simulink model "HyTech_Simulink"  (R2019a)
settings: Solver=ode23t  StartTime=0.0  StopTime=Sch_Cycle(end,1)  RelTol=1e-3  EnableMultiTasking=on
InitFcn:
  | Vehicle_Init_File_L3
StopFcn:
  | Vehicle_Post_File
values from neighbouring files (symbols this model uses):
  Battery_Capacity = 5800/300    (= 19.3333333333)    [Vehicle_Init_File_L3.m]
  Battery_Initial_SOC = 0.9    [Vehicle_Init_File_L3.m]
  Battery_OCV_Data = [3.327826569 3.331337005 3.334822767 3.33828398 3.341720768 3.345133257 3.348521571 3.351885833 3.355226166 3.358542694 3.36183554 3.365104826 ... (412 elements, 1x412)]    [Battery_Data.mat]
  Battery_OCV_SOC_Axis = [0.0004004004004 0.001701701702 0.003003003003 0.004304304304 0.005605605606 0.006906906907 0.008208208208 0.00950950951 0.01081081081 0.01211211211 0.01341341341 0.01471471471 ... (412 elements, 1x412)]    [Battery_Data.mat]
  Battery_OCV_Temp_Axis = [0 10 20 35 55]    [Battery_Data.mat]
  Battery_R_Charge_Data = [1.20043849237 1.12672735687 1.10566703244 1.13725751908 1.18990833015 1.24255914122 1.32680043893 1.43210206107 1.52687352099 0.62127957061 0.5370382729 0.494917624045 ... (45 elements, 9x5)]    [Battery_Data.mat]
  Battery_R_Discharge_Data = [24.63444624 24.49083095 24.34792772 24.20573418 24.06424798 23.92346676 23.78338817 23.64400987 23.5053295 23.36734475 23.23005326 23.09345271 ... (412 elements, 1x412)]    [Battery_Data.mat]
  Battery_R_SOC_Axis = [0.0004004004004 0.001701701702 0.003003003003 0.004304304304 0.005605605606 0.006906906907 0.008208208208 0.00950950951 0.01081081081 0.01211211211 0.01341341341 0.01471471471 ... (412 elements, 1x412)]    [Battery_Data.mat]
  battery_soc_high = 0.9    [Vehicle_Init_File_L3.m]
  battery_soc_low = 0.1    [Vehicle_Init_File_L3.m]
  Front_Sprocket_Teeth = 8    [Vehicle_Init_File_L3.m]
  Logging_Sample_Time_s = 0.01    [Vehicle_Init_File_L3.m]
  Max_Current_Charge = 250    [Vehicle_Init_File_L3.m]
  Max_Current_Discharge = -250    [Vehicle_Init_File_L3.m]
  Rear_Sprocket_Teeth = 41    [Vehicle_Init_File_L3.m]
  Vehicle_Tire_Radius = 0.2286    [Vehicle_Init_File_L3.m]
undefined symbols (not defined in the file or in its folder): Battery_R_Temp_Axis, MG_Eff_Data, MG_Eff_RPM_Axis, MG_Eff_Torque_Axis, MG_Torque_Data, MG_Torque_RPM_Axis, Sch_Cycle
libraries: nesl_utility x12, fl_lib x10, sdl_lib x3, simulink x1
settings Model: Creator=sloghavi3  LastModifiedBy=mweist6
settings SolverCC: SolverResetMethod=Robust
settings DataIOCC: ReturnWorkspaceOutputs=off
settings OptimizationCC: LifeSpan=inf
settings DebuggingCC: PregeneratedLibrarySubsystemCodeDiagnostic=none  SFUnexpectedBacktrackingDiag=warning  SFNoUnconditionalDefaultTransitionDiag=warning  SFExecutionAtInitializationDiag=none  ArithmeticOperatorsInVariantConditions=warning
settings SFSimCC: SimUseLocalCustomCode=off
settings RTWCC: RTWUseLocalCustomCode=off
settings CodeAppCC: StateflowObjectComments=on
settings GRTTargetCC: TargetLangStandard=C89/C90 (ANSI)  GeneratePreprocessorConditionals=Disable all
settings ConfigComp: CovMetricSettings=dw  CovHtmlReporting=on  CovSaveCumulativeToWorkspaceVar=on  CovSaveSingleToWorkspaceVar=on  CovExternalEMLEnable=off
settings SimscapeCC: SimscapeNormalizeSystem=off

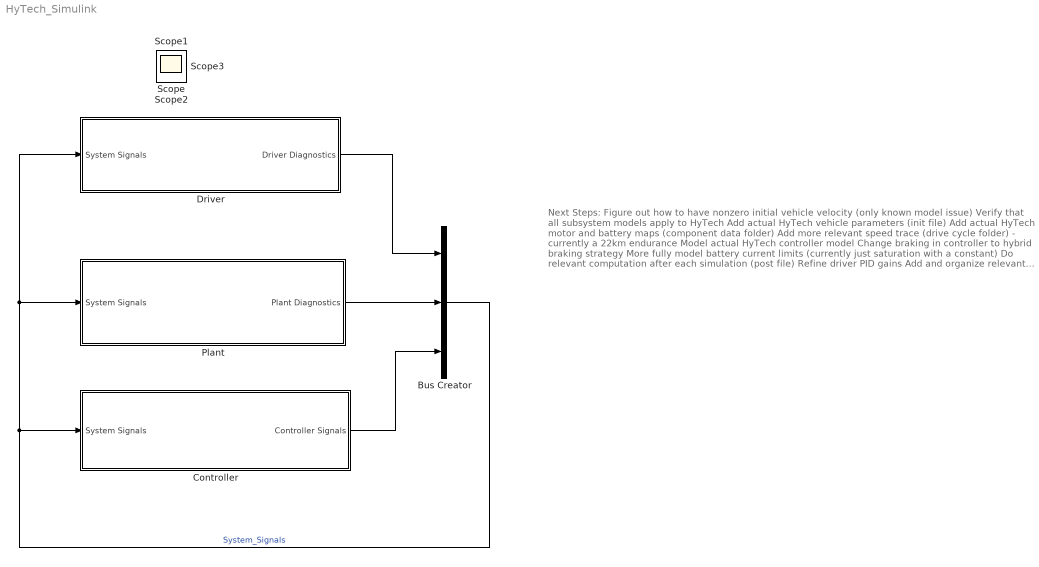
== system HyTech_Simulink ==
  note: Next Steps:
      |
      | Figure out how to have nonzero initial vehicle velocity (only known model issue)
      | Verify that all subsystem models apply to HyTech
      | Add actual HyTech vehicle parameters (init file)
      | Add actual HyTech motor and battery maps (component data folder)
      | Add more relevant speed trace (drive cycle folder) - currently a 22km endurance
      | Model actual HyTech controller model
      | Change braking in controller to hybrid braking strategy
      | More fully model battery current limits (currently just saturation with a constant)
      | Do relevant computation after each simulation (post file)
      | Refine driver PID gains
      | Add and organize relevant scopes in Logging and Visualization subsystem
  Bus Creator : BusCreator  Inputs=3
  Controller : Subsystem
  Driver : Subsystem
  Plant : Subsystem
  Scope{,1..3} (4 alike) : Scope
  wires:
  Driver/1(Driver Diagnostics) -> Bus Creator/1
  Plant/1(Plant Diagnostics) -> Bus Creator/2
  Controller/1(Controller Signals) -> Bus Creator/3
  Bus Creator/1 -> Driver/1(System Signals), Plant/1(System Signals), Controller/1(System Signals)  "System_Signals"

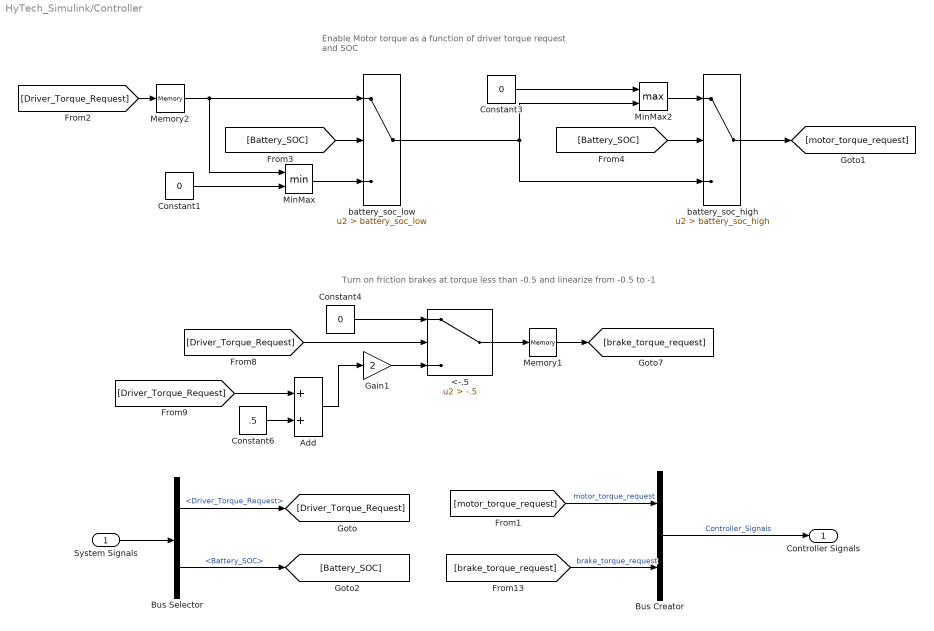
== system HyTech_Simulink/Controller ==
  note: Enable Motor torque as a function of driver torque request
      | and SOC
  note: Turn on friction brakes at torque less than -0.5 and linearize from -0.5 to -1
  System Signals : Inport
  <-.5 : Switch  Criteria=u2 > Threshold  Threshold=-.5
  Add : Sum
  Bus Creator : BusCreator  Inputs=2
  Bus Selector : BusSelector  OutputSignals=Driver_Diagnostics.Driver_Torque_Request,Plant_Diagnostics.Battery_Diagnostics.Battery_SOC
  Constant1 : Constant  Value=0
  Constant3 : Constant  Value=0
  Constant4 : Constant  Value=0
  Constant6 : Constant  Value=.5
  Gain1 : Gain  Gain=2
  Memory1 : Memory
  Memory2 : Memory
  MinMax : MinMax  Inputs=2
  MinMax2 : MinMax  Function=max  Inputs=2
  battery_soc_high : Switch  Criteria=u2 > Threshold  Threshold=battery_soc_high
  battery_soc_low : Switch  Criteria=u2 > Threshold  Threshold=battery_soc_low
  Controller Signals : Outport
  wires:
  Bus Creator/1 -> Controller Signals/1  "Controller_Signals"
  System Signals/1 -> Bus Selector/1
  Bus Selector/1 -> [Driver_Torque_Request]  "<Driver_Torque_Request>"
  [motor_torque_request] -> Bus Creator/1  "motor_torque_request"
  Bus Selector/2 -> [Battery_SOC]  "<Battery_SOC>"
  [Battery_SOC] -> battery_soc_low/2
  [Driver_Torque_Request] -> Memory2/1
  MinMax/1 -> battery_soc_low/3
  [Driver_Torque_Request] -> <-.5/2
  Constant4/1 -> <-.5/1
  [Driver_Torque_Request] -> Add/1
  Constant6/1 -> Add/2
  Add/1 -> Gain1/1
  Gain1/1 -> <-.5/3
  <-.5/1 -> Memory1/1
  [Battery_SOC] -> battery_soc_high/2
  [brake_torque_request] -> Bus Creator/2  "brake_torque_request"
  Memory1/1 -> [brake_torque_request]
  Constant1/1 -> MinMax/2
  battery_soc_low/1 -> battery_soc_high/3, MinMax2/2
  battery_soc_high/1 -> [motor_torque_request]
  Memory2/1 -> MinMax/1, battery_soc_low/1
  MinMax2/1 -> battery_soc_high/1
  Constant3/1 -> MinMax2/1

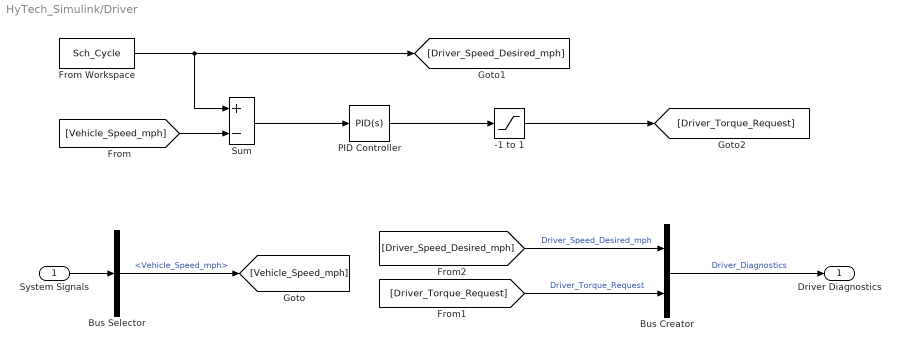
== system HyTech_Simulink/Driver ==
  System Signals : Inport
  -1 to 1 : Saturate  UpperLimit=1  LowerLimit=-1
  Bus Creator : BusCreator  Inputs=2
  Bus Selector : BusSelector  OutputSignals=Plant_Diagnostics.Vehicle_Diagnostics.Vehicle_Speed_mph
  From Workspace : FromWorkspace  VariableName=Sch_Cycle  SampleTime=0
  PID Controller : simulink/Continuous/PID Controller  Controller=PID  Form=Parallel  TimeDomain=Continuous-time  SampleTime=-1  IntegratorMethod=Forward Euler  FilterMethod=Forward Euler  ControllerParametersSource=internal  P=.5  I=.05  D=0.05  UseFilter=on  N=100  TunerSelectOption=Transfer Function Based (PID Tuner App)  InitialConditionSource=internal  InitialConditionForIntegrator=0  InitialConditionForFilter=0  DifferentiatorICPrevScaledInput=0  ExternalReset=none  TrackingMode=off  Kt=1  LimitOutput=off  UpperSaturationLimit=inf  LowerSaturationLimit=-inf  LinearizeAsGain=on  AntiWindupMode=none  Kb=1  POutMin=[]  POutMax=[]  IOutMin=[]  IOutMax=[]  DOutMin=[]  DOutMax=[]  NOutMin=[]  NOutMax=[]  SumOutMin=[]  SumOutMax=[]  SaturationOutMin=[]  SaturationOutMax=[]  PParamMin=[]  PParamMax=[]  IParamMin=[]  IParamMax=[]  DParamMin=[]  DParamMax=[]  NParamMin=[]  NParamMax=[]  KbParamMin=[]  KbParamMax=[]  KtParamMin=[]  KtParamMax=[]  KbOutMin=[]  KbOutMax=[]  KtOutMin=[]  KtOutMax=[]  IntegratorOutMin=[]  IntegratorOutMax=[]  FilterOutMin=[]  FilterOutMax=[]  SumI1OutMin=[]  SumI1OutMax=[]  SumI2OutMin=[]  SumI2OutMax=[]  SumI3OutMin=[]  SumI3OutMax=[]  SumI4OutMin=[]  SumI4OutMax=[]  SumDOutMin=[]  SumDOutMax=[]  DifferentiatorOutMin=[]  DifferentiatorOutMax=[]  FilterDiffOutCoefMin=[]  FilterDiffOutCoefMax=[]  ReciprocalOutMin=[]  ReciprocalOutMax=[]  SumDenOutMin=[]  SumDenOutMax=[]  SumNumOutMin=[]  SumNumOutMax=[]  DivideOutMin=[]  DivideOutMax=[]  IntegratorContinuousStateAttributes=''  IntegratorStateMustResolveToSignalObject=off  IntegratorRTWStateStorageClass=Auto  FilterContinuousStateAttributes=''  FilterStateMustResolveToSignalObject=off  FilterRTWStateStorageClass=Auto  ParallelPVariant=InternalParameters  IdealPVariant=Disabled  IVariant=InternalParameters  DVariant=InternalParameters  IntegratorVariant=Continuous  SatVariant=Disabled  AWVariant=Passthrough  PCopyVariant=Disabled  TRVariant=Disabled  FdbkBlocksVariant=Forward  IdealPFdbkVariant=Disabled  SatFdbkVariant=Disabled  DerivativeFilterVariant=ContFilter  NVariant=InternalParameters  NCopyVariant=Disabled  FilterICVariant=InternalICsFilter  IntegratorICVariant=InternalICs  ExternalResetVariant=Disabled  TRSumVariant=Passthrough  SumFdbkVariant=Disabled  SumVariant=Sum_PID
  Sum : Sum  Inputs=+-
  Driver Diagnostics : Outport
  wires:
  Bus Creator/1 -> Driver Diagnostics/1  "Driver_Diagnostics"
  System Signals/1 -> Bus Selector/1
  Bus Selector/1 -> [Vehicle_Speed_mph]  "<Vehicle_Speed_mph>"
  [Vehicle_Speed_mph] -> Sum/2
  From Workspace/1 -> [Driver_Speed_Desired_mph], Sum/1
  Sum/1 -> PID Controller/1
  PID Controller/1 -> -1 to 1/1
  -1 to 1/1 -> [Driver_Torque_Request]
  [Driver_Torque_Request] -> Bus Creator/2  "Driver_Torque_Request"
  [Driver_Speed_Desired_mph] -> Bus Creator/1  "Driver_Speed_Desired_mph"

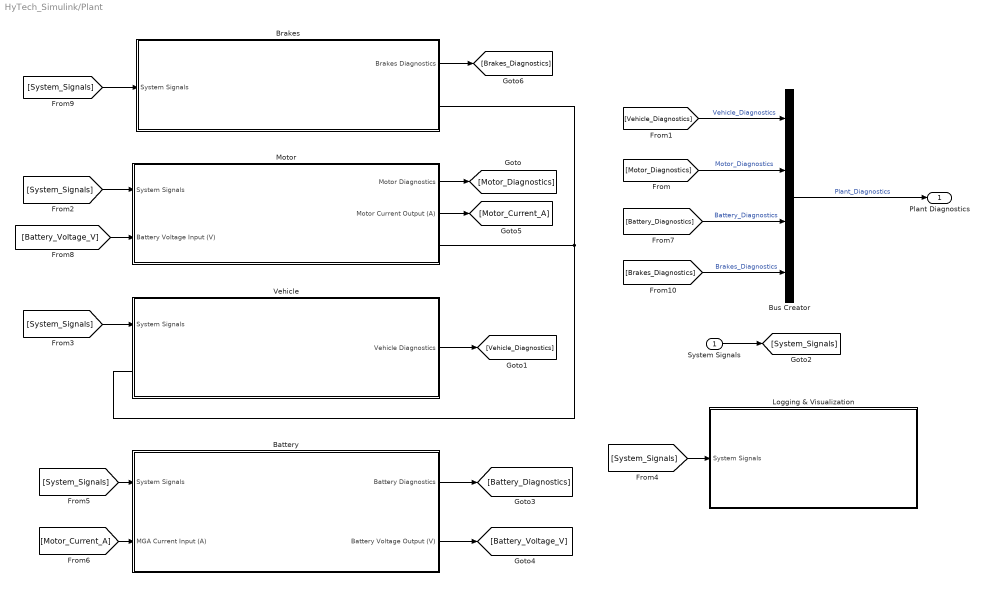
== system HyTech_Simulink/Plant ==
  System Signals : Inport
  Battery : Subsystem
  Brakes : Subsystem
  Bus Creator : BusCreator  Inputs=4
  Logging & Visualization : Subsystem
  Motor : Subsystem
  Vehicle : Subsystem
  Plant Diagnostics : Outport
  wires:
  Bus Creator/1 -> Plant Diagnostics/1  "Plant_Diagnostics"
  System Signals/1 -> [System_Signals]
  Motor/1(Motor Diagnostics) -> [Motor_Diagnostics]
  [Motor_Diagnostics] -> Bus Creator/2  "Motor_Diagnostics"
  [Vehicle_Diagnostics] -> Bus Creator/1  "Vehicle_Diagnostics"
  [System_Signals] -> Motor/1(System Signals)
  [System_Signals] -> Vehicle/1(System Signals)
  [System_Signals] -> Logging & Visualization/1(System Signals)
  [System_Signals] -> Battery/1(System Signals)
  Battery/2("Battery Voltage Output (V) ") -> [Battery_Voltage_V]
  Battery/1("Battery Diagnostics ") -> [Battery_Diagnostics]
  [Motor_Current_A] -> Battery/2("MGA Current Input (A) ")
  [Battery_Diagnostics] -> Bus Creator/3  "Battery_Diagnostics"
  Vehicle/1(Vehicle Diagnostics) -> [Vehicle_Diagnostics]
  [Battery_Voltage_V] -> Motor/2("Battery Voltage Input (V) ")
  Motor/2("Motor Current Output (A) ") -> [Motor_Current_A]
  [System_Signals] -> Brakes/1(System Signals)
  Brakes/1(Brakes Diagnostics) -> [Brakes_Diagnostics]
  [Brakes_Diagnostics] -> Bus Creator/4  "Brakes_Diagnostics"
  connections:
  Brakes/RConn1 -- Vehicle/LConn1 -- Motor/RConn1

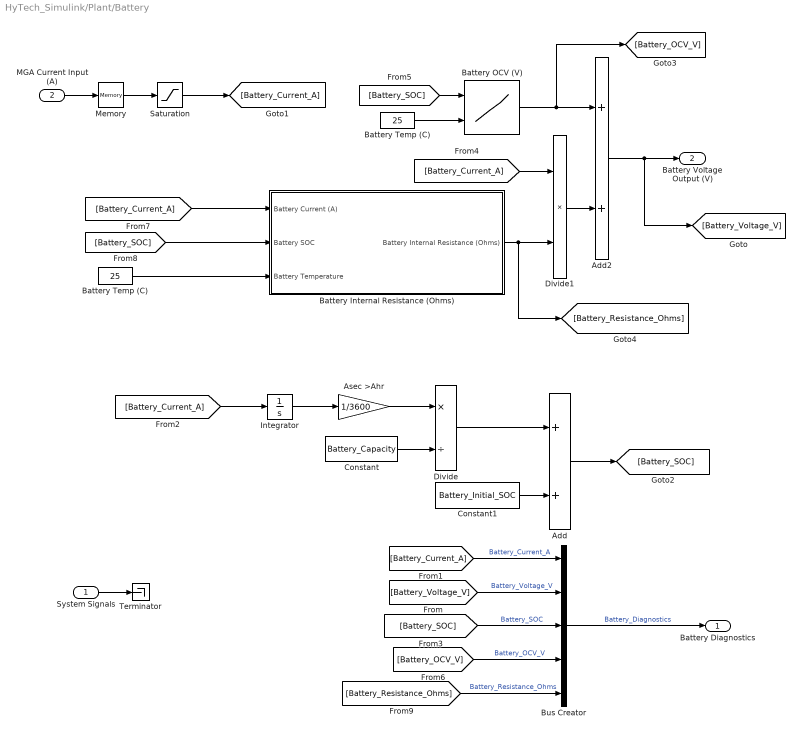
== system HyTech_Simulink/Plant/Battery ==
  System Signals : Inport
  "MGA Current Input (A) " : Inport  Port=2
  Add : Sum
  Add2 : Sum
  Asec >Ahr : Gain  Gain=1/3600
  "Battery Internal Resistance (Ohms) " : Subsystem
  Battery OCV (V) : Lookup_n-D  BreakpointsForDimension1=Battery_OCV_SOC_Axis  BreakpointsForDimension2=Battery_OCV_Temp_Axis  Table=Battery_OCV_Data  InternalRulePriority=Speed  RndMeth=Simplest  InputSameDT=on
  Battery Temp (C) : Constant  Value=25
  "Battery Temp (C) " : Constant  Value=25
  Bus Creator : BusCreator  Inputs=5
  Constant : Constant  Value=Battery_Capacity
  Constant1 : Constant  Value=Battery_Initial_SOC
  Divide : Product  Inputs=*/
  Divide1 : Product  Inputs=**
  Integrator : Integrator
  Memory : Memory
  Saturation : Saturate  UpperLimit=Max_Current_Charge  LowerLimit=Max_Current_Discharge
  Terminator : Terminator
  "Battery Diagnostics " : Outport
  "Battery Voltage Output (V) " : Outport  Port=2
  wires:
  System Signals/1 -> Terminator/1
  Bus Creator/1 -> "Battery Diagnostics "/1  "Battery_Diagnostics"
  [Battery_Voltage_V] -> Bus Creator/2  "Battery_Voltage_V"
  [Battery_Current_A] -> Bus Creator/1  "Battery_Current_A"
  [Battery_Current_A] -> Integrator/1
  Integrator/1 -> Asec >Ahr/1
  Asec >Ahr/1 -> Divide/1
  Constant/1 -> Divide/2
  Constant1/1 -> Add/2
  Divide/1 -> Add/1
  Add/1 -> [Battery_SOC]
  [Battery_SOC] -> Bus Creator/3  "Battery_SOC"
  "MGA Current Input (A) "/1 -> Memory/1
  [Battery_Current_A] -> Divide1/1
  Divide1/1 -> Add2/2
  Add2/1 -> [Battery_Voltage_V], "Battery Voltage Output (V) "/1
  Battery OCV (V)/1 -> [Battery_OCV_V], Add2/1
  "Battery Temp (C) "/1 -> Battery OCV (V)/2
  [Battery_SOC] -> Battery OCV (V)/1
  [Battery_OCV_V] -> Bus Creator/4  "Battery_OCV_V"
  "Battery Internal Resistance (Ohms) "/1("Battery Internal Resistance (Ohms) ") -> [Battery_Resistance_Ohms], Divide1/2
  [Battery_Current_A] -> "Battery Internal Resistance (Ohms) "/1(Battery Current (A))
  [Battery_SOC] -> "Battery Internal Resistance (Ohms) "/2(Battery SOC)
  Battery Temp (C)/1 -> "Battery Internal Resistance (Ohms) "/3("Battery Temperature ")
  [Battery_Resistance_Ohms] -> Bus Creator/5  "Battery_Resistance_Ohms"
  Memory/1 -> Saturation/1
  Saturation/1 -> [Battery_Current_A]

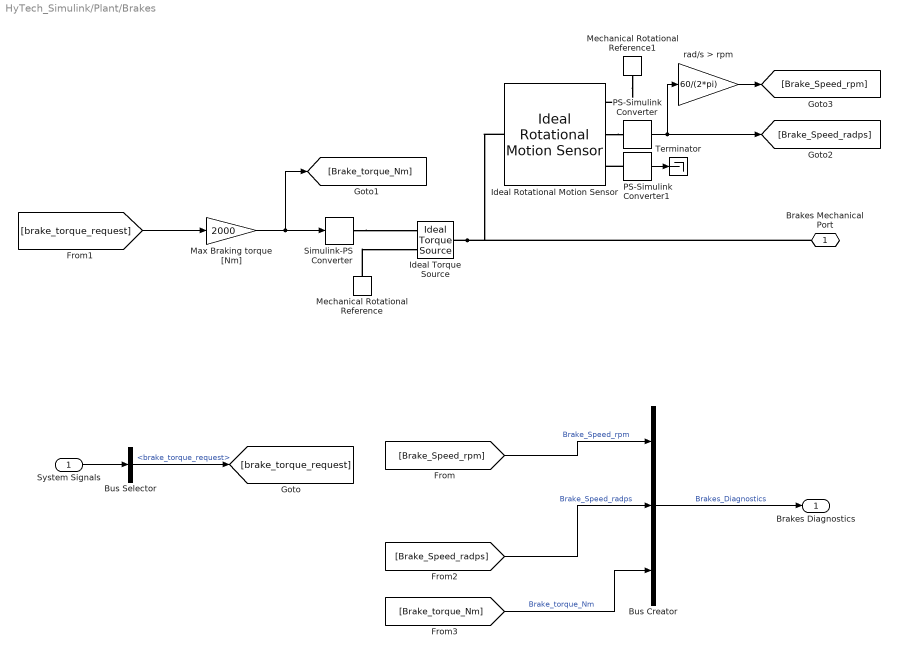
== system HyTech_Simulink/Plant/Brakes ==
  System Signals : Inport
  Bus Creator : BusCreator  Inputs=3
  Bus Selector : BusSelector  OutputSignals=Controller_Signals.brake_torque_request
  Ideal Rotational Motion Sensor : fl_lib/Mechanical/Mechanical Sensors/Ideal Rotational Motion Sensor  offset=0 rad
  Ideal Torque Source : fl_lib/Mechanical/Mechanical Sources/Ideal Torque Source
  Max Braking torque [Nm] : Gain  Gain=2000
  Mechanical Rotational Reference : fl_lib/Mechanical/Rotational Elements/Mechanical Rotational Reference
  Mechanical Rotational Reference1 : fl_lib/Mechanical/Rotational Elements/Mechanical Rotational Reference
  PS-Simulink Converter : nesl_utility/PS-Simulink Converter  PhysicalDomain=network_engine_domain  SubClassName=ps_output  LeftPortType=input  RightPortType=output  PseudoPeriodic=off  Frequencies=[]  Unit=1  AffineConversion=off
  PS-Simulink Converter1 : nesl_utility/PS-Simulink Converter  PhysicalDomain=network_engine_domain  SubClassName=ps_output  LeftPortType=input  RightPortType=output  PseudoPeriodic=off  Frequencies=[]  Unit=1  AffineConversion=off
  Simulink-PS Converter : nesl_utility/Simulink-PS Converter  PhysicalDomain=network_engine_domain  SubClassName=ps_input  LeftPortType=input  RightPortType=output  PseudoPeriodic=off  Frequencies=[]  NoiseDistribution=none  NoiseParameters=[]  Unit=1  AffineConversion=off  FilteringAndDerivatives=zero  SimscapeFilterOrder=2  InputFilterTimeConstant=0.01  UdotUserProvided=1
  Terminator : Terminator
  rad/s > rpm : Gain  Gain=60/(2*pi)
  Brakes Mechanical Port : PMIOPort  Side=Right
  Brakes Diagnostics : Outport
  wires:
  PS-Simulink Converter/1 -> rad/s > rpm/1, [Brake_Speed_radps]
  System Signals/1 -> Bus Selector/1
  PS-Simulink Converter1/1 -> Terminator/1
  rad/s > rpm/1 -> [Brake_Speed_rpm]
  Bus Selector/1 -> [brake_torque_request]  "<brake_torque_request>"
  [brake_torque_request] -> Max Braking torque [Nm]/1
  Bus Creator/1 -> Brakes Diagnostics/1  "Brakes_Diagnostics"
  [Brake_Speed_rpm] -> Bus Creator/1  "Brake_Speed_rpm"
  [Brake_Speed_radps] -> Bus Creator/2  "Brake_Speed_radps"
  Max Braking torque [Nm]/1 -> [Brake_torque_Nm], Simulink-PS Converter/1
  [Brake_torque_Nm] -> Bus Creator/3  "Brake_torque_Nm"
  connections:
  Ideal Torque Source/LConn1 -- Brakes Mechanical Port/RConn1 -- Ideal Rotational Motion Sensor/LConn1
  Simulink-PS Converter/RConn1 -- Ideal Torque Source/RConn1
  Mechanical Rotational Reference/LConn1 -- Ideal Torque Source/RConn2
  PS-Simulink Converter1/LConn1 -- Ideal Rotational Motion Sensor/RConn3
  Mechanical Rotational Reference1/LConn1 -- Ideal Rotational Motion Sensor/RConn1
  Ideal Rotational Motion Sensor/RConn2 -- PS-Simulink Converter/LConn1

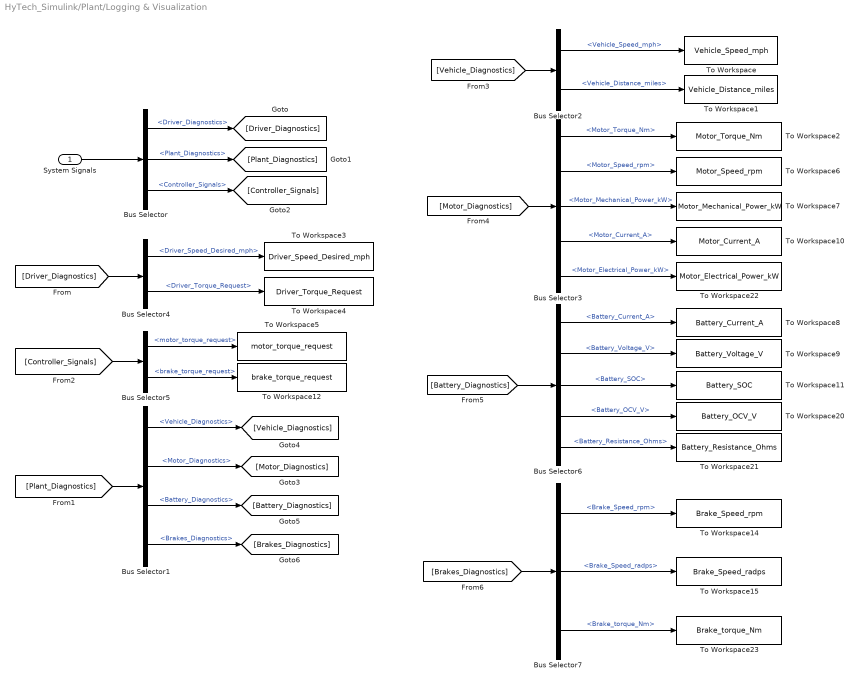
== system HyTech_Simulink/Plant/Logging & Visualization ==
  System Signals : Inport
  Bus Selector : BusSelector  OutputSignals=Driver_Diagnostics,Plant_Diagnostics,Controller_Signals
  Bus Selector1 : BusSelector  OutputSignals=Vehicle_Diagnostics,Motor_Diagnostics,Battery_Diagnostics,Brakes_Diagnostics
  Bus Selector2 : BusSelector  OutputSignals=Vehicle_Speed_mph,Vehicle_Distance_miles
  Bus Selector3 : BusSelector  OutputSignals=Motor_Torque_Nm,Motor_Speed_rpm,Motor_Mechanical_Power_kW,Motor_Current_A,Motor_Electrical_Power_kW
  Bus Selector4 : BusSelector  OutputSignals=Driver_Speed_Desired_mph,Driver_Torque_Request
  Bus Selector5 : BusSelector  OutputSignals=motor_torque_request,brake_torque_request
  Bus Selector6 : BusSelector  OutputSignals=Battery_Current_A,Battery_Voltage_V,Battery_SOC,Battery_OCV_V,Battery_Resistance_Ohms
  Bus Selector7 : BusSelector  OutputSignals=Brake_Speed_rpm,Brake_Speed_radps,Brake_torque_Nm
  To Workspace : ToWorkspace  VariableName=Vehicle_Speed_mph  SampleTime=Logging_Sample_Time_s
  To Workspace1 : ToWorkspace  VariableName=Vehicle_Distance_miles  SampleTime=Logging_Sample_Time_s
  To Workspace10 : ToWorkspace  VariableName=Motor_Current_A  SampleTime=Logging_Sample_Time_s
  To Workspace11 : ToWorkspace  VariableName=Battery_SOC  SampleTime=Logging_Sample_Time_s
  To Workspace12 : ToWorkspace  VariableName=brake_torque_request  SampleTime=Logging_Sample_Time_s
  To Workspace14 : ToWorkspace  VariableName=Brake_Speed_rpm  SampleTime=Logging_Sample_Time_s
  To Workspace15 : ToWorkspace  VariableName=Brake_Speed_radps  SampleTime=Logging_Sample_Time_s
  To Workspace2 : ToWorkspace  VariableName=Motor_Torque_Nm  SampleTime=Logging_Sample_Time_s
  To Workspace20 : ToWorkspace  VariableName=Battery_OCV_V  SampleTime=Logging_Sample_Time_s
  To Workspace21 : ToWorkspace  VariableName=Battery_Resistance_Ohms  SampleTime=Logging_Sample_Time_s
  To Workspace22 : ToWorkspace  VariableName=Motor_Electrical_Power_kW  SampleTime=Logging_Sample_Time_s
  To Workspace23 : ToWorkspace  VariableName=Brake_torque_Nm  SampleTime=Logging_Sample_Time_s
  To Workspace3 : ToWorkspace  VariableName=Driver_Speed_Desired_mph  SampleTime=Logging_Sample_Time_s
  To Workspace4 : ToWorkspace  VariableName=Driver_Torque_Request  SampleTime=Logging_Sample_Time_s
  To Workspace5 : ToWorkspace  VariableName=motor_torque_request  SampleTime=Logging_Sample_Time_s
  To Workspace6 : ToWorkspace  VariableName=Motor_Speed_rpm  SampleTime=Logging_Sample_Time_s
  To Workspace7 : ToWorkspace  VariableName=Motor_Mechanical_Power_kW  SampleTime=Logging_Sample_Time_s
  To Workspace8 : ToWorkspace  VariableName=Battery_Current_A  SampleTime=Logging_Sample_Time_s
  To Workspace9 : ToWorkspace  VariableName=Battery_Voltage_V  SampleTime=Logging_Sample_Time_s
  wires:
  System Signals/1 -> Bus Selector/1
  Bus Selector/1 -> [Driver_Diagnostics]  "<Driver_Diagnostics>"
  Bus Selector/2 -> [Plant_Diagnostics]  "<Plant_Diagnostics>"
  Bus Selector/3 -> [Controller_Signals]  "<Controller_Signals>"
  [Driver_Diagnostics] -> Bus Selector4/1
  [Controller_Signals] -> Bus Selector5/1
  [Plant_Diagnostics] -> Bus Selector1/1
  Bus Selector1/2 -> [Motor_Diagnostics]  "<Motor_Diagnostics>"
  Bus Selector1/1 -> [Vehicle_Diagnostics]  "<Vehicle_Diagnostics>"
  [Vehicle_Diagnostics] -> Bus Selector2/1
  [Motor_Diagnostics] -> Bus Selector3/1
  Bus Selector2/1 -> To Workspace/1  "<Vehicle_Speed_mph>"
  Bus Selector3/1 -> To Workspace2/1  "<Motor_Torque_Nm>"
  Bus Selector4/1 -> To Workspace3/1  "<Driver_Speed_Desired_mph>"
  Bus Selector4/2 -> To Workspace4/1  "<Driver_Torque_Request>"
  Bus Selector5/1 -> To Workspace5/1  "<motor_torque_request>"
  Bus Selector3/2 -> To Workspace6/1  "<Motor_Speed_rpm>"
  Bus Selector3/3 -> To Workspace7/1  "<Motor_Mechanical_Power_kW>"
  Bus Selector1/3 -> [Battery_Diagnostics]  "<Battery_Diagnostics>"
  [Battery_Diagnostics] -> Bus Selector6/1
  Bus Selector6/1 -> To Workspace8/1  "<Battery_Current_A>"
  Bus Selector6/2 -> To Workspace9/1  "<Battery_Voltage_V>"
  Bus Selector3/4 -> To Workspace10/1  "<Motor_Current_A>"
  Bus Selector6/3 -> To Workspace11/1  "<Battery_SOC>"
  Bus Selector6/4 -> To Workspace20/1  "<Battery_OCV_V>"
  Bus Selector6/5 -> To Workspace21/1  "<Battery_Resistance_Ohms>"
  Bus Selector3/5 -> To Workspace22/1  "<Motor_Electrical_Power_kW>"
  Bus Selector1/4 -> [Brakes_Diagnostics]  "<Brakes_Diagnostics>"
  [Brakes_Diagnostics] -> Bus Selector7/1
  Bus Selector7/1 -> To Workspace14/1  "<Brake_Speed_rpm>"
  Bus Selector7/2 -> To Workspace15/1  "<Brake_Speed_radps>"
  Bus Selector7/3 -> To Workspace23/1  "<Brake_torque_Nm>"
  Bus Selector2/2 -> To Workspace1/1  "<Vehicle_Distance_miles>"
  Bus Selector5/2 -> To Workspace12/1  "<brake_torque_request>"

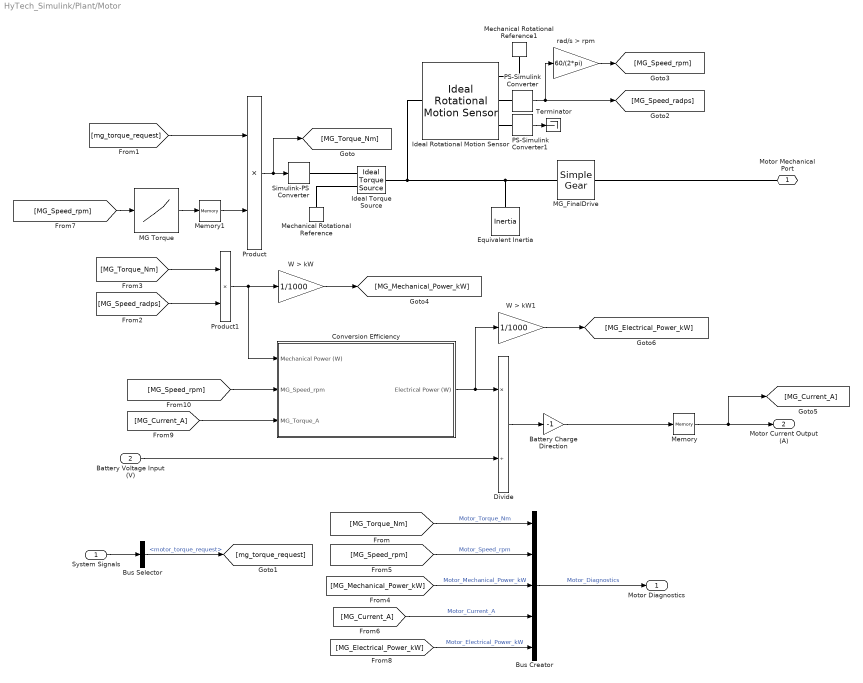
== system HyTech_Simulink/Plant/Motor ==
  System Signals : Inport
  "Battery Voltage Input (V) " : Inport  Port=2
  Battery Charge Direction : Gain  Gain=-1
  Bus Creator : BusCreator  Inputs=5
  Bus Selector : BusSelector  OutputSignals=Controller_Signals.motor_torque_request
  Conversion Efficiency : Subsystem
  Divide : Product  Inputs=*/
  Equivalent Inertia : fl_lib/Mechanical/Rotational Elements/Inertia  inertia=Equivalent_Drivetrain_Inertia kg*m^2  w_specify=off  w_priority=High  w=0 rad/s  w_nominal_specify=off  w_nominal_unit=rad/s  w_nominal_value=1  t_specify=off  t_priority=None  t=0 N*m  t_nominal_specify=off  t_nominal_unit=N*m  t_nominal_value=1
  Ideal Rotational Motion Sensor : fl_lib/Mechanical/Mechanical Sensors/Ideal Rotational Motion Sensor  offset=0 rad
  Ideal Torque Source : fl_lib/Mechanical/Mechanical Sources/Ideal Torque Source
  MG Torque : Lookup_n-D  NumberOfTableDimensions=1  BreakpointsForDimension1=MG_Torque_RPM_Axis  Table=MG_Torque_Data  InternalRulePriority=Speed  RndMeth=Simplest  InputSameDT=on
  MG_FinalDrive : sdl_lib/Gears/Simple Gear  ratio=Rear_Sprocket_Teeth / Front_Sprocket_Teeth  rotation_direction=1  friction_model=1  T_noload=0.1 N*m  T_nom=5 N*m  efficiency_nom=0.8  efficiency=0.8  mu_visc=[0.0, 0.0] N*m/(rad/s)  w_thr=0.01 rad/s  pwr_thr=0.001 W  enable_faults=simscape.enum.onoff.off  efficiency_fault=0.05  external_fault=simscape.enum.onoff.off  temporal_fault=simscape.enum.onoff.off  fault_time=5 s  fault_angles=pi / 12 rad  report_fault=1  temperature_TLU=[280.0, 300.0, 320.0] K  load_TLU=[1.0, 5.0, 10.0] N*m  efficiency_TLU=[0.95, 0.9, 0.85]  efficiency_TLU2=[0.85, 0.8, 0.75; 0.95, 0.9, 0.85; 0.85, 0.8, 0.7]  thermal_mass=50 J/K  T_init=300 K
      settings: SourceProductName=Simscape Driveline
  Mechanical Rotational Reference : fl_lib/Mechanical/Rotational Elements/Mechanical Rotational Reference
  Mechanical Rotational Reference1 : fl_lib/Mechanical/Rotational Elements/Mechanical Rotational Reference
  Memory : Memory
  Memory1 : Memory
  PS-Simulink Converter : nesl_utility/PS-Simulink Converter  PhysicalDomain=network_engine_domain  SubClassName=ps_output  LeftPortType=input  RightPortType=output  PseudoPeriodic=off  Frequencies=[]  Unit=1  AffineConversion=off
  PS-Simulink Converter1 : nesl_utility/PS-Simulink Converter  PhysicalDomain=network_engine_domain  SubClassName=ps_output  LeftPortType=input  RightPortType=output  PseudoPeriodic=off  Frequencies=[]  Unit=1  AffineConversion=off
  Product : Product
  Product1 : Product
  Simulink-PS Converter : nesl_utility/Simulink-PS Converter  PhysicalDomain=network_engine_domain  SubClassName=ps_input  LeftPortType=input  RightPortType=output  PseudoPeriodic=off  Frequencies=[]  NoiseDistribution=none  NoiseParameters=[]  Unit=1  AffineConversion=off  FilteringAndDerivatives=zero  SimscapeFilterOrder=2  InputFilterTimeConstant=0.01  UdotUserProvided=1
  Terminator : Terminator
  W > kW : Gain  Gain=1/1000
  W > kW1 : Gain  Gain=1/1000
  rad/s > rpm : Gain  Gain=60/(2*pi)
  Motor Mechanical Port : PMIOPort  Side=Right
  Motor Diagnostics : Outport
  "Motor Current Output (A) " : Outport  Port=2
  wires:
  Bus Creator/1 -> Motor Diagnostics/1  "Motor_Diagnostics"
  [MG_Torque_Nm] -> Bus Creator/1  "Motor_Torque_Nm"
  System Signals/1 -> Bus Selector/1
  Bus Selector/1 -> [mg_torque_request]  "<motor_torque_request>"
  MG Torque/1 -> Memory1/1
  Product/1 -> [MG_Torque_Nm], Simulink-PS Converter/1
  [mg_torque_request] -> Product/1
  PS-Simulink Converter1/1 -> Terminator/1
  PS-Simulink Converter/1 -> rad/s > rpm/1, [MG_Speed_radps]
  rad/s > rpm/1 -> [MG_Speed_rpm]
  Product1/1 -> Conversion Efficiency/1("Mechanical Power (W) "), W > kW/1
  [MG_Speed_radps] -> Product1/2
  [MG_Torque_Nm] -> Product1/1
  W > kW/1 -> [MG_Mechanical_Power_kW]
  [MG_Mechanical_Power_kW] -> Bus Creator/3  "Motor_Mechanical_Power_kW"
  [MG_Speed_rpm] -> Bus Creator/2  "Motor_Speed_rpm"
  Divide/1 -> Battery Charge Direction/1
  [MG_Current_A] -> Bus Creator/4  "Motor_Current_A"
  "Battery Voltage Input (V) "/1 -> Divide/2
  [MG_Speed_rpm] -> MG Torque/1
  Conversion Efficiency/1(Electrical Power (W)) -> W > kW1/1, Divide/1
  W > kW1/1 -> [MG_Electrical_Power_kW]
  [MG_Electrical_Power_kW] -> Bus Creator/5  "Motor_Electrical_Power_kW"
  [MG_Current_A] -> Conversion Efficiency/3(MG_Torque_A)
  [MG_Speed_rpm] -> Conversion Efficiency/2(MG_Speed_rpm)
  Memory/1 -> [MG_Current_A], "Motor Current Output (A) "/1
  Memory1/1 -> Product/2
  Battery Charge Direction/1 -> Memory/1
  connections:
  Simulink-PS Converter/RConn1 -- Ideal Torque Source/RConn1
  Equivalent Inertia/LConn1 -- MG_FinalDrive/LConn1 -- Ideal Rotational Motion Sensor/LConn1 -- Ideal Torque Source/LConn1
  Mechanical Rotational Reference/LConn1 -- Ideal Torque Source/RConn2
  Ideal Rotational Motion Sensor/RConn2 -- PS-Simulink Converter/LConn1
  Mechanical Rotational Reference1/LConn1 -- Ideal Rotational Motion Sensor/RConn1
  PS-Simulink Converter1/LConn1 -- Ideal Rotational Motion Sensor/RConn3
  MG_FinalDrive/RConn1 -- Motor Mechanical Port/RConn1

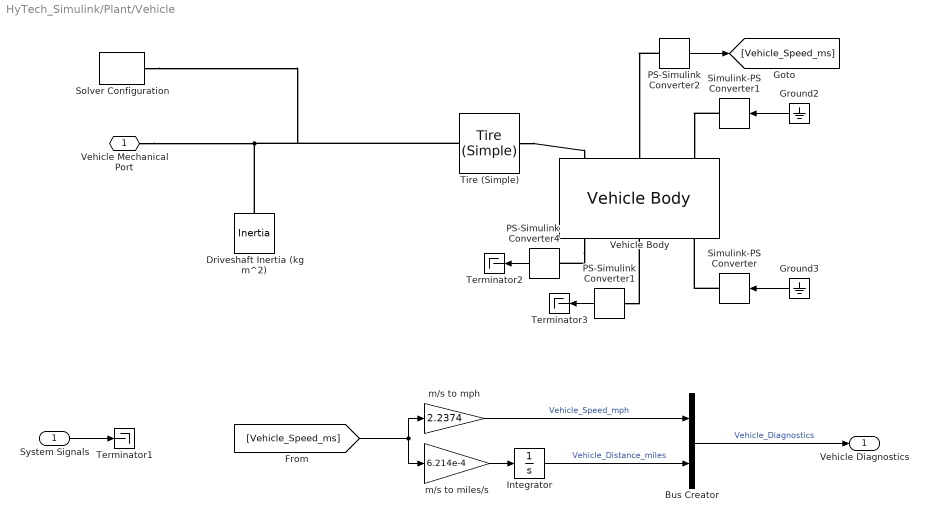
== system HyTech_Simulink/Plant/Vehicle ==
  System Signals : Inport
  Bus Creator : BusCreator  Inputs=2
  "Driveshaft Inertia (kg m^2) " : fl_lib/Mechanical/Rotational Elements/Inertia  inertia=Vehicle_DShaft_Inertia kg*m^2  w_specify=off  w_priority=High  w=0 rad/s  w_nominal_specify=off  w_nominal_unit=rad/s  w_nominal_value=1  t_specify=off  t_priority=None  t=0 N*m  t_nominal_specify=off  t_nominal_unit=N*m  t_nominal_value=1
  Ground2 : Ground
  Ground3 : Ground
  Integrator : Integrator
  PS-Simulink Converter1 : nesl_utility/PS-Simulink Converter  PhysicalDomain=network_engine_domain  SubClassName=ps_output  LeftPortType=input  RightPortType=output  PseudoPeriodic=off  Frequencies=[]  Unit=1  AffineConversion=off
  PS-Simulink Converter2 : nesl_utility/PS-Simulink Converter  PhysicalDomain=network_engine_domain  SubClassName=ps_output  LeftPortType=input  RightPortType=output  PseudoPeriodic=off  Frequencies=[]  Unit=1  AffineConversion=off
  PS-Simulink Converter4 : nesl_utility/PS-Simulink Converter  PhysicalDomain=network_engine_domain  SubClassName=ps_output  LeftPortType=input  RightPortType=output  PseudoPeriodic=off  Frequencies=[]  Unit=1  AffineConversion=off
  Simulink-PS Converter : nesl_utility/Simulink-PS Converter  PhysicalDomain=network_engine_domain  SubClassName=ps_input  LeftPortType=input  RightPortType=output  PseudoPeriodic=off  Frequencies=[]  NoiseDistribution=none  NoiseParameters=[]  Unit=1  AffineConversion=off  FilteringAndDerivatives=zero  SimscapeFilterOrder=1  InputFilterTimeConstant=0.001  UdotUserProvided=1
  Simulink-PS Converter1 : nesl_utility/Simulink-PS Converter  PhysicalDomain=network_engine_domain  SubClassName=ps_input  LeftPortType=input  RightPortType=output  PseudoPeriodic=off  Frequencies=[]  NoiseDistribution=none  NoiseParameters=[]  Unit=1  AffineConversion=off  FilteringAndDerivatives=zero  SimscapeFilterOrder=1  InputFilterTimeConstant=0.001  UdotUserProvided=1
  Solver Configuration : nesl_utility/Solver Configuration  PhysicalDomain=network_engine_domain  SubClassName=solver  LeftPortType=input  RightPortType=generic  Tones=[]  Harmonics=[]  SimulateNoise=off  Profile=off  UseLocalSampling=off  EnableSwitchedLinearOptims=on  FrequencyDomain=off  UseCCode=off  RelTol=0.001  AbsTol=1e-06  MinStep=1e-09  ToWorkspace=off  RevertToSquareIcSolve=off  NumHomotopyIterations=100  PhasorMode=off  PhasorModeNumHarmonics=1  DoDC=off  ResidualTolerance=1e-09  UseLocalSolver=off  LocalSolverChoice=NE_BACKWARD_EULER_ADVANCER  LocalSolverSampleTime=0.001  DoFixedCost=off  MaxNonlinIter=3  MaxModeIter=2  LinearAlgebra=Sparse  EquationFormulation=NE_TIME_EF  DelaysMemoryBudget=1024  AutomaticFiltering=on  FilteringTimeConstant=0.001  PartitionStorageMethod=AS_NEEDED  PartitionMemoryBudget=1024  PartitionMethod=FAST
  Terminator1 : Terminator
  Terminator2 : Terminator
  Terminator3 : Terminator
  Tire (Simple) : sdl_lib/Tires & Vehicles/Tire (Simple)  r_tire=Vehicle_Tire_Radius m  model_compliance=0  stiffness=1e6 N/m  damping=1000 N/(m/s)  model_inertia=1  tire_inertia=Wheel_Plus_Tire_Inertia kg*m^2  initial_velocity=Sch_Cycle(1,2)*0.44704/Vehicle_Tire_Radius rad/s
      settings: SourceProductName=Simscape Driveline  SourceProductBaseCode=LD
  Vehicle Body : sdl_lib/Tires & Vehicles/Vehicle Body  mass=Vehicle_Mass kg  n_w=2  x_f=Vehicle_FrontToCG_in in  x_r=Vehicle_RearToCG_in in  y_c=Vehicle_CG_in in  mass_var=simscape.enum.onoff.off  model_pitch=0  inertia=4000 kg*m^2  suspension_model=1  k_f=1e4 N/m  b_f=1e4 N/(m/s)  k_r=1e4 N/m  b_r=1e4 N/(m/s)  k_f_TLU=[-2000, -1000, 0, 1000, 2000] N  x_f_TLU=[-.4, -.2, 0, .2, .4] m  b_f_TLU=[-200, -100, 0, 100, 200] N  v_f_TLU=[-4, -2, 0, 2, 4] m/s  k_r_TLU=[-2000, -1000, 0, 1000, 2000] N  x_r_TLU=[-.4, -.2, 0, .2, .4] m  b_r_TLU=[-200, -100, 0, 100, 200] N  v_r_TLU=[-4, -2, 0, 2, 4] m/s  interp_method=simscape.enum.interpolation.linear  extrap_method=simscape.enum.extrapolation.linear  model_hardstop=0  upper_bound_f=.25 m  lower_bound_f=-.25 m  stop_k_f=1e6 N/m  stop_b_f=150 N/(m/s)  upper_bound_r=.25 m  lower_bound_r=-.25 m  stop_k_r=1e6 N/m  stop_b_r=150 N/(m/s)  initial_pitch=0 rad  initial_pitch_rate=0 rad/s  g=9.81 m/s^2  liftoff_warning=0  area=Vehicle_Frontal_Area m^2  Cd=Vehicle_Cd  rho=1.225 kg/m^3  v_specify=on  v_priority=High  v=Sch_Cycle(1,2)/2.2374 m/s  v_nominal_specify=off  v_nominal_unit=m/s  v_nominal_value=1
      settings: SourceProductName=Simscape Driveline
  m/s to miles/s : Gain  Gain=6.214e-4
  m/s to mph : Gain  Gain=2.2374
  Vehicle Mechanical Port : PMIOPort  Side=Left
  Vehicle Diagnostics : Outport
  wires:
  Bus Creator/1 -> Vehicle Diagnostics/1  "Vehicle_Diagnostics"
  Ground2/1 -> Simulink-PS Converter1/1
  Ground3/1 -> Simulink-PS Converter/1
  PS-Simulink Converter1/1 -> Terminator3/1
  PS-Simulink Converter2/1 -> [Vehicle_Speed_ms]
  [Vehicle_Speed_ms] -> m/s to mph/1, m/s to miles/s/1
  m/s to miles/s/1 -> Integrator/1
  Integrator/1 -> Bus Creator/2  "Vehicle_Distance_miles"
  m/s to mph/1 -> Bus Creator/1  "Vehicle_Speed_mph"
  System Signals/1 -> Terminator1/1
  PS-Simulink Converter4/1 -> Terminator2/1
  connections:
  Vehicle Mechanical Port/RConn1 -- Tire (Simple)/LConn1 -- Solver Configuration/RConn1 -- "Driveshaft Inertia (kg m^2) "/LConn1
  Tire (Simple)/RConn1 -- Vehicle Body/LConn1
  Simulink-PS Converter1/RConn1 -- Vehicle Body/LConn3
  Simulink-PS Converter/RConn1 -- Vehicle Body/RConn3
  PS-Simulink Converter1/LConn1 -- Vehicle Body/RConn2
  PS-Simulink Converter2/LConn1 -- Vehicle Body/LConn2
  Vehicle Body/RConn1 -- PS-Simulink Converter4/LConn1

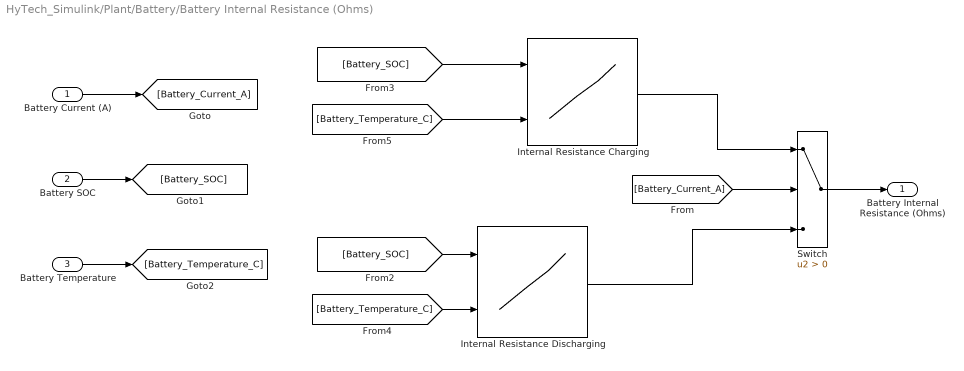
== system HyTech_Simulink/Plant/Battery/Battery Internal Resistance (Ohms)  ==
  Battery Current (A) : Inport
  Battery SOC : Inport  Port=2
  "Battery Temperature " : Inport  Port=3
  Internal Resistance Charging : Lookup_n-D  BreakpointsForDimension1=Battery_R_SOC_Axis  BreakpointsForDimension2=Battery_R_Temp_Axis  Table=Battery_R_Charge_Data  InternalRulePriority=Speed  RndMeth=Simplest  InputSameDT=on
  Internal Resistance Discharging : Lookup_n-D  BreakpointsForDimension1=Battery_R_SOC_Axis  BreakpointsForDimension2=Battery_R_Temp_Axis  Table=Battery_R_Discharge_Data  InternalRulePriority=Speed  RndMeth=Simplest  InputSameDT=on
  Switch : Switch  Criteria=u2 > Threshold
  "Battery Internal Resistance (Ohms) " : Outport
  wires:
  Battery Current (A)/1 -> [Battery_Current_A]
  Battery SOC/1 -> [Battery_SOC]
  "Battery Temperature "/1 -> [Battery_Temperature_C]
  [Battery_Current_A] -> Switch/2
  [Battery_Temperature_C] -> Internal Resistance Discharging/2
  [Battery_Temperature_C] -> Internal Resistance Charging/2
  [Battery_SOC] -> Internal Resistance Discharging/1
  [Battery_SOC] -> Internal Resistance Charging/1
  Switch/1 -> "Battery Internal Resistance (Ohms) "/1
  Internal Resistance Charging/1 -> Switch/1
  Internal Resistance Discharging/1 -> Switch/3

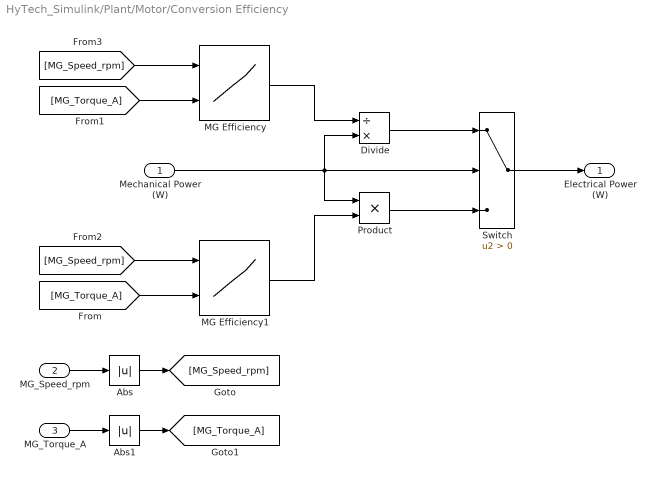
== system HyTech_Simulink/Plant/Motor/Conversion Efficiency ==
  "Mechanical Power (W) " : Inport
  MG_Speed_rpm : Inport  Port=2
  MG_Torque_A : Inport  Port=3
  Abs : Abs
  Abs1 : Abs
  Divide : Product  Inputs=/*
  MG Efficiency : Lookup_n-D  BreakpointsForDimension1=MG_Eff_RPM_Axis  BreakpointsForDimension2=MG_Eff_Torque_Axis  Table=MG_Eff_Data  InternalRulePriority=Speed  RndMeth=Simplest  InputSameDT=on
  MG Efficiency1 : Lookup_n-D  BreakpointsForDimension1=MG_Eff_RPM_Axis  BreakpointsForDimension2=MG_Eff_Torque_Axis  Table=MG_Eff_Data  InternalRulePriority=Speed  RndMeth=Simplest  InputSameDT=on
  Product : Product
  Switch : Switch  Criteria=u2 > Threshold
  Electrical Power (W) : Outport
  wires:
  Switch/1 -> Electrical Power (W)/1
  "Mechanical Power (W) "/1 -> Product/1, Divide/2, Switch/2
  MG Efficiency1/1 -> Product/2
  Divide/1 -> Switch/1
  Product/1 -> Switch/3
  MG Efficiency/1 -> Divide/1
  MG_Speed_rpm/1 -> Abs/1
  MG_Torque_A/1 -> Abs1/1
  [MG_Torque_A] -> MG Efficiency1/2
  [MG_Torque_A] -> MG Efficiency/2
  [MG_Speed_rpm] -> MG Efficiency1/1
  [MG_Speed_rpm] -> MG Efficiency/1
  Abs/1 -> [MG_Speed_rpm]
  Abs1/1 -> [MG_Torque_A]
